simulink model "Motor_Model"  (Simulink 7.5)
settings: Solver=ode45  StartTime=0.0  StopTime=10.0  RelTol=1e-3
undefined symbols (not defined in the file or in its folder): b, J, K, L, R
settings Model: Creator=maen  LastModifiedBy=Rick

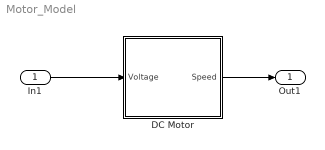
== system Motor_Model ==
  In1 : Inport  OutDataType=fixdt(1, 16)  OutScaling=2^0
  DC Motor : Subsystem
  Out1 : Outport  OutDataType=fixdt(1, 16)  OutScaling=2^0
  wires:
  In1/1 -> DC Motor/1(Voltage)
  DC Motor/1(" Speed") -> Out1/1

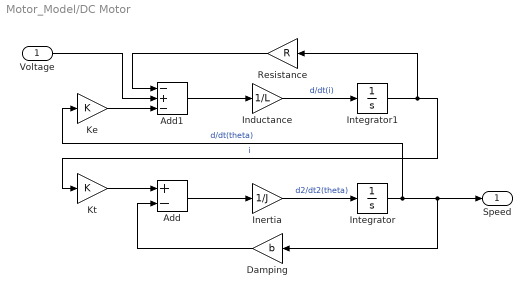
== system Motor_Model/DC Motor ==
  Voltage : Inport  OutDataType=fixdt(1, 16)  OutScaling=2^0
  Add : Sum  Inputs=+-  OutDataType=fixdt(1, 16)  OutScaling=2^-10
  Add1 : Sum  Inputs=-+-  OutDataType=fixdt(1, 16)  OutScaling=2^-10
  Damping : Gain  Gain=b  ParameterDataType=fixdt(1, 16)  ParameterScaling=2^0  OutDataType=fixdt(1, 16)  OutScaling=2^0
  Inductance : Gain  Gain=1/L  ParameterDataType=fixdt(1, 16)  ParameterScaling=2^0  OutDataType=fixdt(1, 16)  OutScaling=2^0
  Inertia : Gain  Gain=1/J  ParameterDataType=fixdt(1, 16)  ParameterScaling=2^0  OutDataType=fixdt(1, 16)  OutScaling=2^0
  Integrator : Integrator
  Integrator1 : Integrator
  Ke : Gain  Gain=K  ParameterDataType=fixdt(1, 16)  ParameterScaling=2^0  OutDataType=fixdt(1, 16)  OutScaling=2^0
  Kt : Gain  Gain=K  ParameterDataType=fixdt(1, 16)  ParameterScaling=2^0  OutDataType=fixdt(1, 16)  OutScaling=2^0
  Resistance : Gain  Gain=R  ParameterDataType=fixdt(1, 16)  ParameterScaling=2^0  OutDataType=fixdt(1, 16)  OutScaling=2^0
  " Speed" : Outport  OutDataType=fixdt(1, 16)  OutScaling=2^0
  wires:
  Integrator1/1 -> Kt/1, Resistance/1  "i"
  Inductance/1 -> Integrator1/1  "d/dt(i)"
  Inertia/1 -> Integrator/1  "d2/dt2(theta)"
  Integrator/1 -> Ke/1, Damping/1, " Speed"/1  "d/dt(theta)"
  Add1/1 -> Inductance/1
  Add/1 -> Inertia/1
  Damping/1 -> Add/2
  Kt/1 -> Add/1
  Resistance/1 -> Add1/1
  Ke/1 -> Add1/3
  Voltage/1 -> Add1/2
